simulink model "on_slope_harness_real"  (R2017b)
settings: Solver=VariableStepAuto  StartTime=0.0  StopTime=300  RelTol=1e-3
undefined symbols (not defined in the file): sigbuilder_block
settings Model: Creator=Kris  LastModifiedBy=Kris

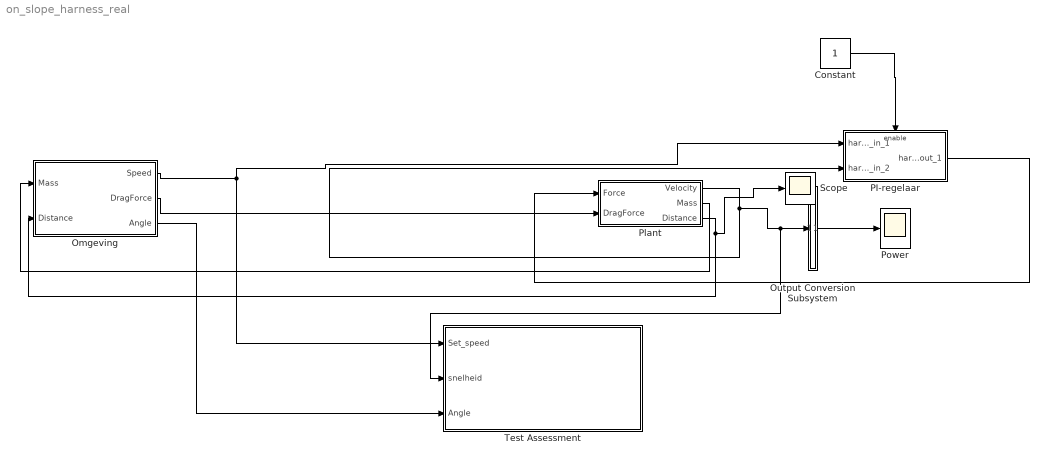
== system on_slope_harness_real ==
  Constant : Constant
  Omgeving : Subsystem
  Output Conversion Subsystem : Subsystem  Tag=__SLT_OCS__  Description=|
      | Signal spec.
      | and routing
      settings: AttributesFormatString=%<Description>
  "PI-regelaar " : Subsystem  Tag=__SL_testing_harness_stub_
  Plant : Subsystem
  Power : Scope
  Scope : Scope
  Test Assessment : Test Sequence  TreatAsAtomicUnit=on
  wires:
  Output Conversion Subsystem/1(Outport_1) -> Power/1
  "PI-regelaar "/1(harness_out_1) -> Plant/1("Force ")
  Constant/1 -> "PI-regelaar "/Enable
  Plant/1(Velocity) -> "PI-regelaar "/2(harness_in_2), Test Assessment/2(snelheid), Output Conversion Subsystem/1(Inport_1)
  Omgeving/1(Speed) -> "PI-regelaar "/1(harness_in_1), Test Assessment/1(Set_speed)
  Plant/2(Mass) -> Omgeving/1(Mass)
  Plant/3(Distance) -> Scope/1, Omgeving/2(Distance)
  Omgeving/2(DragForce) -> Plant/2(DragForce)
  Omgeving/3(Angle) -> Test Assessment/3(Angle)

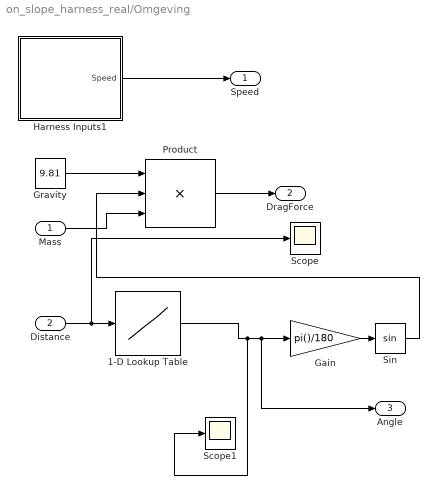
== system on_slope_harness_real/Omgeving ==
  Mass : Inport
  Distance : Inport  Port=2
  1-D Lookup Table : Lookup_n-D  NumberOfTableDimensions=1  BreakpointsSpecification=Even spacing  BreakpointsForDimension1=[0:100000]  Table=(20*sin([0:(60000)]/2000+60))  InternalRulePriority=Speed  RndMeth=Simplest  InputSameDT=on
  Gain : Gain  Gain=pi()/180
  Gravity : Constant  Value=9.81
  Harness Inputs1 : Subsystem  Tag=STV Subsys  LoadFcn=sigbuilder_block('load');  StartFcn=sigbuilder_block('start');  StopFcn=sigbuilder_block('stop');  ClipboardFcn=sigbuilder_block('clipboard');  mask(Sigbuilder block){tuvar=[0:10]}
      mask init:
      | if ~strcmp(get_param(bdroot(gcb),'SimulationStatus'),'stopped'),tuvar = sigbuilder_block('maskInit'); end
      settings: CopyFcn=sigbuilder_block('copy');  DeleteFcn=sigbuilder_block('delete');  ModelCloseFcn=sigbuilder_block('modelClose');  PreSaveFcn=sigbuilder_block('preSave');  PauseFcn=sigbuilder_block('pause');  ContinueFcn=sigbuilder_block('continue');  NameChangeFcn=sigbuilder_block('namechange');  OpenFcn=sigbuilder_block('open',[263.25 43.5 735.75 399.75 ]);  CloseFcn=sigbuilder_block('close');
      mask Display: plot(0, 0, 100, 100,[2, 2, 32, 32, 2], [68, 8, 8, 68, 68],[32, 2], [38, 38], [32, 19, 2],[53, 60, 44], [32, 17, 17, 2],[16, 16, 31, 31]);txt = getActiveGroup(gcbh);text(2, 100, txt,'verticalAlignment', 'top');
  Product : Product  Inputs=3
  Scope : Scope
  Scope1 : Scope
  Sin : Trigonometry
  Speed : Outport
  DragForce : Outport  Port=2
  Angle : Outport  Port=3
  wires:
  1-D Lookup Table/1 -> Angle/1, Gain/1, Scope1/1
  Mass/1 -> Product/3
  Product/1 -> DragForce/1
  Distance/1 -> Scope/1, 1-D Lookup Table/1
  Harness Inputs1/1(Speed) -> Speed/1
  Gravity/1 -> Product/1
  Sin/1 -> Product/2
  Gain/1 -> Sin/1

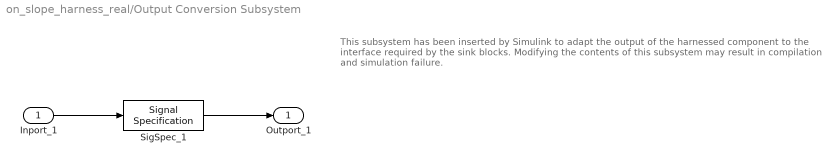
== system on_slope_harness_real/Output Conversion Subsystem ==
  note: This subsystem has been inserted by Simulink to adapt the output of the harnessed component to the interface required by the sink blocks.
      |  Modifying the contents of this subsystem may result in compilation and simulation failure.
  Inport_1 : Inport
  SigSpec_1 : SignalSpecification  OutDataTypeStr=double  Dimensions=[1]
  Outport_1 : Outport
  wires:
  Inport_1/1 -> SigSpec_1/1
  SigSpec_1/1 -> Outport_1/1

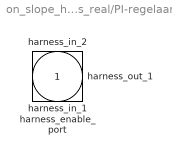
== system on_slope_harness_real/PI-regelaar  ==
  harness_in_1 : Inport
  harness_in_2 : Inport  Port=2
  harness_enable_port : EnablePort
  harness_out_1 : Outport

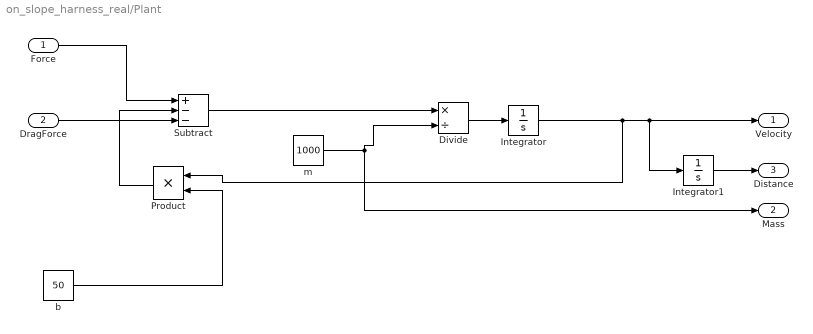
== system on_slope_harness_real/Plant ==
  "Force " : Inport
  DragForce : Inport  Port=2
  Divide : Product  Inputs=*/
  Integrator : Integrator
  Integrator1 : Integrator
  Product : Product
  Subtract : Sum  Inputs=+--
  b : Constant  Value=50
  m : Constant  Value=1000
  Velocity : Outport
  Mass : Outport  Port=2
  Distance : Outport  Port=3
  wires:
  Product/1 -> Subtract/2
  b/1 -> Product/2
  Subtract/1 -> Divide/1
  "Force "/1 -> Subtract/1
  Divide/1 -> Integrator/1
  m/1 -> Divide/2, Mass/1
  DragForce/1 -> Subtract/3
  Integrator1/1 -> Distance/1
  Integrator/1 -> Product/1, Velocity/1, Integrator1/1

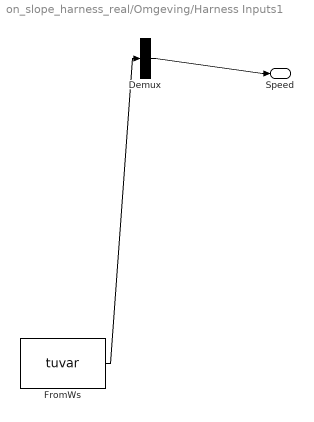
== system on_slope_harness_real/Omgeving/Harness Inputs1 ==
  Demux : Demux  Tag=STV Demux  Outputs=1
  FromWs : FromWorkspace  Tag=STV FromWs  VariableName=tuvar  SampleTime=0
      SigBuilderData=|
      | dataSet.timeRange = [0 180]
      | dataSet.name = 'Group 1'
      | sbobj.Name = 'Signal Builder'
      | sbobj.Groups.Name = 'Group 1'
      | sbobj.Groups.Signals.Name = 'Speed'
      | sbobj.Groups.Signals.XData = [0 180]
      | sbobj.Groups.Signals.YData = [30 30]
      | sbobj.Groups.TimeRange = [0 180]
  Speed : Outport  Tag=STV Outport
  wires:
  FromWs/1 -> Demux/1
  Demux/1 -> Speed/1

== stateflow chart on_slope_harness_real/Test Assessment ==
  settings: stateMachineType=SIMPLIFIED_MACHINE
  state InitializeTest
    state step_1_1
      verify(Set_speed > (snelheid - 1.4));
      verify(Set_speed < (snelheid +1.4));
    state step_1_2
    (default) -> (junction 22)
    InitializeTest -> (junction 22) [order 1]
    (junction 22) -> (junction 23) [order 1] : [t > 10 && Angle > -20 && Angle <20
        | ]
    (junction 23) -> step_1_1 [order 1] : [~in(step_1_1)]
    (junction 22) -> (junction 56) [order 2]
    (junction 23) -> (junction 26) [order 2]
    (junction 56) -> (junction 57)
    (junction 57) -> step_1_2 [order 1] : [~in(step_1_2)]
    (junction 57) -> (junction 60) [order 2]
  state WaitStabilize
  (default) -> InitializeTest
  InitializeTest -> WaitStabilize [order 1] : [hasChanged(Set_speed)
      | ]
  WaitStabilize -> InitializeTest : [after(10,sec)
      | ]
  data: Set_speed input; snelheid input; speedtocheck local; speed local; Angle input
